simulink library "r2daq_blocks"  (R2012b)
settings: Solver=ode45  StartTime=0.0  StopTime=10.0  RelTol=1e-3
undefined symbols (not defined in the file or in its folder): biquad_iir, feedback_iir, filters, libddc, sfp, synth, xlfir_8x16
libraries: xbsIndex_r4 x4088, casper_library_misc x21, dspsigops x16, casper_library_delays x10, xps_library x1
(part 4 of 23)

== system r2daq_blocks/DigitalDownConverterExt/bus_mul_sine ==
  a : Inport
  b : Inport  Port=2
  a*b_bussify : Subsystem  AncestorBlock=casper_library_flow_control/bus_create  mask(bus_create){inputNum=16}
      mask prompts: inputNum "Number of inputs:"
      mask init:
      | bus_create_init(gcb,...
      |     'inputNum', inputNum);
  a_debus : Subsystem  AncestorBlock=casper_library_flow_control/bus_expand  mask(bus_expand){mode=divisions of arbitrary size, outputNum=1, outputWidth=[8 8 8 8 8 8 8 8 8 8 8 8 8 8 8 8], outputBinaryPt=[7 7 7 7 7 7 7 7 7 7 7 7 7 7 7 7], outputArithmeticType=[1 1 1 1 1 1 1 1 1 1 1 1 1 1 1 1], show_format=on, outputToWorkspace=off, variablePrefix=, outputToModelAsWell=on}
      mask prompts: outputNum "Number of outputs:"; outputWidth "Output width [msb ... lsb]:"; outputBinaryPt "Output binary point position [msb ... lsb]:"; outputArithmeticType "Output arithmetic type (ufix=0, fix=1, bool=2) [msb ... lsb]:"; show_format "Print format string?"; outputToWorkspace "Output to workspace?"; variablePrefix "Variable name prefix:"; outputToModelAsWell "Output to model as well?"
      mask help:
      | Expands a 'bus' made using a bus_create or Xilinx
      | concat block.
      | The input will be divided into the specified number
      | of outputs with the specified arithmetic types.
      | Divisions are made from most significant bit.
      mask init: same as r2daq_blocks/DigitalDownConverterExt/bus_mul_cosine/a_debus
      settings: AttributesFormatString=16 outputs: f8.7,f8.7,f8.7,f8.7,f8.7,f8.7,f8.7,f8.7,f8.7,f8.7,f8.7,f8.7,f8.7,f8.7,f8.7,f8.7,
      mask TypeOptions mode: divisions of equal size | divisions of arbitrary size
      mask Callback mode: bus_expand_callback();
      mask Callback outputWidth: bus_expand_callback();
      mask Callback outputToWorkspace: bus_expand_callback();
  b_debus : Subsystem  AncestorBlock=casper_library_flow_control/bus_expand  mask(bus_expand){mode=divisions of arbitrary size, outputNum=1, outputWidth=[11 11 11 11 11 11 11 11 11 11 11 11 11 11 11 11], outputBinaryPt=[9 9 9 9 9 9 9 9 9 9 9 9 9 9 9 9], outputArithmeticType=[1 1 1 1 1 1 1 1 1 1 1 1 1 1 1 1], show_format=on, outputToWorkspace=off, variablePrefix=, outputToModelAsWell=on}
      mask prompts: outputNum "Number of outputs:"; outputWidth "Output width [msb ... lsb]:"; outputBinaryPt "Output binary point position [msb ... lsb]:"; outputArithmeticType "Output arithmetic type (ufix=0, fix=1, bool=2) [msb ... lsb]:"; show_format "Print format string?"; outputToWorkspace "Output to workspace?"; variablePrefix "Variable name prefix:"; outputToModelAsWell "Output to model as well?"
      mask help:
      | Expands a 'bus' made using a bus_create or Xilinx
      | concat block.
      | The input will be divided into the specified number
      | of outputs with the specified arithmetic types.
      | Divisions are made from most significant bit.
      mask init: same as r2daq_blocks/DigitalDownConverterExt/bus_mul_cosine/a_debus
      settings: AttributesFormatString=16 outputs: f11.9,f11.9,f11.9,f11.9,f11.9,f11.9,f11.9,f11.9,f11.9,f11.9,f11.9,f11.9,f11.9,f11.9,f11.9,f11.9,
      mask TypeOptions mode: divisions of equal size | divisions of arbitrary size
      mask Callback mode: bus_expand_callback();
      mask Callback outputWidth: bus_expand_callback();
      mask Callback outputToWorkspace: bus_expand_callback();
  mult{1..16} (16 alike) : xbsIndex_r4/Mult  precision=User Defined  arith_type="Signed  (2's comp)"  n_bits=18  bin_pt=16  quantization=Truncate  overflow=Wrap  en=off  latency=mult_latency  dbl_ovrd=off  use_behavioral_HDL=on  opt=Speed  use_embedded=off  optimum_pipeline=off  pipeline=on  use_rpm=on  placement_style=Triangular  block_type=mult
  repa : Subsystem  AncestorBlock=casper_library_bus/bus_replicate  mask(bus_replicate){replication=1, latency=0, misc=off, implementation=core}
      mask prompts: replication "replication factor"; misc "misc support"; implementation "delay implementation"
      mask help: Output bus formed by replicating input bus a number of times
      mask init:
      | bus_replicate_init(gcb, ...
      |     'replication', replication, ...
      |     'latency', latency, ...
      |     'implementation', implementation, ...
      |     'misc', misc);
      mask TypeOptions implementation: core | behavioral
  repb : Subsystem  AncestorBlock=casper_library_bus/bus_replicate  mask(bus_replicate){replication=1, latency=0, misc=off, implementation=core}
      mask prompts: replication "replication factor"; misc "misc support"; implementation "delay implementation"
      mask help: Output bus formed by replicating input bus a number of times
      mask init:
      | bus_replicate_init(gcb, ...
      |     'replication', replication, ...
      |     'latency', latency, ...
      |     'implementation', implementation, ...
      |     'misc', misc);
      mask TypeOptions implementation: core | behavioral
  a*b : Outport
  wires:
  a/1 -> repa/1(in)
  b/1 -> repb/1(in)
  repa/1(out) -> a_debus/1(bus_in)
  repb/1(out) -> b_debus/1(bus_in)
  a_debus/1(msb_out16) -> mult1/1
  b_debus/1(msb_out16) -> mult1/2
  a_debus/2(out15) -> mult2/1
  b_debus/2(out15) -> mult2/2
  a_debus/3(out14) -> mult3/1
  b_debus/3(out14) -> mult3/2
  a_debus/4(out13) -> mult4/1
  b_debus/4(out13) -> mult4/2
  a_debus/5(out12) -> mult5/1
  b_debus/5(out12) -> mult5/2
  a_debus/6(out11) -> mult6/1
  b_debus/6(out11) -> mult6/2
  a_debus/7(out10) -> mult7/1
  b_debus/7(out10) -> mult7/2
  a_debus/8(out9) -> mult8/1
  b_debus/8(out9) -> mult8/2
  a_debus/9(out8) -> mult9/1
  b_debus/9(out8) -> mult9/2
  a_debus/10(out7) -> mult10/1
  b_debus/10(out7) -> mult10/2
  a_debus/11(out6) -> mult11/1
  b_debus/11(out6) -> mult11/2
  a_debus/12(out5) -> mult12/1
  b_debus/12(out5) -> mult12/2
  a_debus/13(out4) -> mult13/1
  b_debus/13(out4) -> mult13/2
  a_debus/14(out3) -> mult14/1
  b_debus/14(out3) -> mult14/2
  a_debus/15(out2) -> mult15/1
  b_debus/15(out2) -> mult15/2
  a_debus/16(lsb_out1) -> mult16/1
  b_debus/16(lsb_out1) -> mult16/2
  mult1/1 -> a*b_bussify/1(in1)
  mult2/1 -> a*b_bussify/2(in2)
  mult3/1 -> a*b_bussify/3(in3)
  mult4/1 -> a*b_bussify/4(in4)
  mult5/1 -> a*b_bussify/5(in5)
  mult6/1 -> a*b_bussify/6(in6)
  mult7/1 -> a*b_bussify/7(in7)
  mult8/1 -> a*b_bussify/8(in8)
  mult9/1 -> a*b_bussify/9(in9)
  mult10/1 -> a*b_bussify/10(in10)
  mult11/1 -> a*b_bussify/11(in11)
  mult12/1 -> a*b_bussify/12(in12)
  mult13/1 -> a*b_bussify/13(in13)
  mult14/1 -> a*b_bussify/14(in14)
  mult15/1 -> a*b_bussify/15(in15)
  mult16/1 -> a*b_bussify/16(in16)
  a*b_bussify/1(bus_out) -> a*b/1

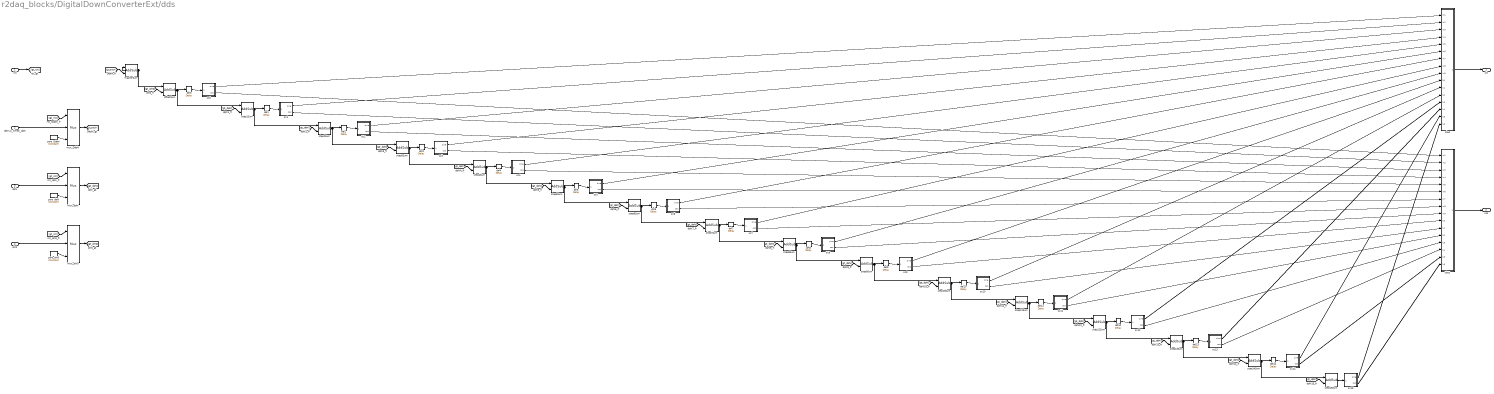
== system r2daq_blocks/DigitalDownConverterExt/dds ==
  rst : Inport
  demux_times_dphi : Inport  Port=2
  dphi : Inport  Port=3
  phi0 : Inport  Port=4
  cbus : Subsystem  AncestorBlock=casper_library_flow_control/bus_create  mask(bus_create){inputNum=16}
      mask prompts: inputNum "Number of inputs:"
      mask init:
      | bus_create_init(gcb,...
      |     'inputNum', inputNum);
  del0 : xbsIndex_r4/Delay  rst=off  infoeditControl=Selection of Reset will increase slice count due to use of real FFs and instead of SRLs  en=off  latency=15  dbl_ovrd=off  reg_retiming=off  block_type=delay
  del1 : xbsIndex_r4/Delay  rst=off  infoeditControl=Selection of Reset will increase slice count due to use of real FFs and instead of SRLs  en=off  latency=14  dbl_ovrd=off  reg_retiming=off  block_type=delay
  del10 : xbsIndex_r4/Delay  rst=off  infoeditControl=Selection of Reset will increase slice count due to use of real FFs and instead of SRLs  en=off  latency=5  dbl_ovrd=off  reg_retiming=off  block_type=delay
  del11 : xbsIndex_r4/Delay  rst=off  infoeditControl=Selection of Reset will increase slice count due to use of real FFs and instead of SRLs  en=off  latency=4  dbl_ovrd=off  reg_retiming=off  block_type=delay
  del12 : xbsIndex_r4/Delay  rst=off  infoeditControl=Selection of Reset will increase slice count due to use of real FFs and instead of SRLs  en=off  latency=3  dbl_ovrd=off  reg_retiming=off  block_type=delay
  del13 : xbsIndex_r4/Delay  rst=off  infoeditControl=Selection of Reset will increase slice count due to use of real FFs and instead of SRLs  en=off  latency=2  dbl_ovrd=off  reg_retiming=off  block_type=delay
  del14 : xbsIndex_r4/Delay  rst=off  infoeditControl=Selection of Reset will increase slice count due to use of real FFs and instead of SRLs  en=off  latency=1  dbl_ovrd=off  reg_retiming=off  block_type=delay
  del2 : xbsIndex_r4/Delay  rst=off  infoeditControl=Selection of Reset will increase slice count due to use of real FFs and instead of SRLs  en=off  latency=13  dbl_ovrd=off  reg_retiming=off  block_type=delay
  del3 : xbsIndex_r4/Delay  rst=off  infoeditControl=Selection of Reset will increase slice count due to use of real FFs and instead of SRLs  en=off  latency=12  dbl_ovrd=off  reg_retiming=off  block_type=delay
  del4 : xbsIndex_r4/Delay  rst=off  infoeditControl=Selection of Reset will increase slice count due to use of real FFs and instead of SRLs  en=off  latency=11  dbl_ovrd=off  reg_retiming=off  block_type=delay
  del5 : xbsIndex_r4/Delay  rst=off  infoeditControl=Selection of Reset will increase slice count due to use of real FFs and instead of SRLs  en=off  latency=10  dbl_ovrd=off  reg_retiming=off  block_type=delay
  del6 : xbsIndex_r4/Delay  rst=off  infoeditControl=Selection of Reset will increase slice count due to use of real FFs and instead of SRLs  en=off  latency=9  dbl_ovrd=off  reg_retiming=off  block_type=delay
  del7 : xbsIndex_r4/Delay  rst=off  infoeditControl=Selection of Reset will increase slice count due to use of real FFs and instead of SRLs  en=off  latency=8  dbl_ovrd=off  reg_retiming=off  block_type=delay
  del8 : xbsIndex_r4/Delay  rst=off  infoeditControl=Selection of Reset will increase slice count due to use of real FFs and instead of SRLs  en=off  latency=7  dbl_ovrd=off  reg_retiming=off  block_type=delay
  del9 : xbsIndex_r4/Delay  rst=off  infoeditControl=Selection of Reset will increase slice count due to use of real FFs and instead of SRLs  en=off  latency=6  dbl_ovrd=off  reg_retiming=off  block_type=delay
  masterSum : xbsIndex_r4/AddSub  mode=Addition  use_carryin=off  use_carryout=off  en=off  latency=1  precision=User Defined  arith_type=Unsigned  n_bits=10  bin_pt=0  quantization=Truncate  overflow=Wrap  dbl_ovrd=off  use_behavioral_HDL=off  hw_selection=Fabric  pipelined=off  block_type=addsub
  mux_Ddphi : xbsIndex_r4/Mux  inputs=2  en=off  latency=0  precision=Full  arith_type=Unsigned  n_bits=16  bin_pt=14  quantization=Truncate  overflow=Wrap  dbl_ovrd=off  block_type=mux
  mux_dphi : xbsIndex_r4/Mux  inputs=2  en=off  latency=0  precision=Full  arith_type=Unsigned  n_bits=16  bin_pt=14  quantization=Truncate  overflow=Wrap  dbl_ovrd=off  block_type=mux
  mux_phi0 : xbsIndex_r4/Mux  inputs=2  en=off  latency=0  precision=Full  arith_type=Unsigned  n_bits=16  bin_pt=14  quantization=Truncate  overflow=Wrap  dbl_ovrd=off  block_type=mux
  offsetSum : xbsIndex_r4/AddSub  mode=Addition  use_carryin=off  use_carryout=off  en=off  latency=1  precision=User Defined  arith_type=Unsigned  n_bits=10  bin_pt=0  quantization=Truncate  overflow=Wrap  dbl_ovrd=off  use_behavioral_HDL=off  hw_selection=Fabric  pipelined=off  block_type=addsub
  sbus : Subsystem  AncestorBlock=casper_library_flow_control/bus_create  mask(bus_create){inputNum=16}
      mask prompts: inputNum "Number of inputs:"
      mask init:
      | bus_create_init(gcb,...
      |     'inputNum', inputNum);
  sc0 : Subsystem  Tag=casper:sincos  AncestorBlock=casper_library_downconverter/sincos  mask(sincos){func=sine and cosine, neg_sin=off, neg_cos=off, symmetric=on, handle_sync=off, depth_bits=10, bit_width=11, bram_latency=2}
      mask prompts: func "Function"; neg_sin "Negative sine"; neg_cos "Negative cosine"; symmetric "Symmetric output"; handle_sync "Handle sync"; depth_bits "Lookup table depth (2^?)"; bit_width "Output bit width"; bram_latency "BRAM latency"
      mask init:
      | sincos_init(gcb, ...
      |     'func', func, ...
      |     'neg_sin', neg_sin, ...
      |     'neg_cos', neg_cos, ...
      |     'symmetric', symmetric, ...
      |     'handle_sync', handle_sync, ...
      |     'depth_bits', depth_bits, ...
      |     'bit_width', bit_width, ...
      |     'bram_latency', bram_latency);
      mask TypeOptions func: cosine | sine | sine and cosine
  sc1 : Subsystem  Tag=casper:sincos  AncestorBlock=casper_library_downconverter/sincos  mask(sincos){func=sine and cosine, neg_sin=off, neg_cos=off, symmetric=on, handle_sync=off, depth_bits=10, bit_width=11, bram_latency=2}
      mask prompts: func "Function"; neg_sin "Negative sine"; neg_cos "Negative cosine"; symmetric "Symmetric output"; handle_sync "Handle sync"; depth_bits "Lookup table depth (2^?)"; bit_width "Output bit width"; bram_latency "BRAM latency"
      mask init: same as r2daq_blocks/DigitalDownConverterExt/dds/sc0
      mask TypeOptions func: cosine | sine | sine and cosine
  sc10 : Subsystem  Tag=casper:sincos  AncestorBlock=casper_library_downconverter/sincos  mask(sincos){func=sine and cosine, neg_sin=off, neg_cos=off, symmetric=on, handle_sync=off, depth_bits=10, bit_width=11, bram_latency=2}
      mask prompts: func "Function"; neg_sin "Negative sine"; neg_cos "Negative cosine"; symmetric "Symmetric output"; handle_sync "Handle sync"; depth_bits "Lookup table depth (2^?)"; bit_width "Output bit width"; bram_latency "BRAM latency"
      mask init: same as r2daq_blocks/DigitalDownConverterExt/dds/sc0
      mask TypeOptions func: cosine | sine | sine and cosine
  sc11 : Subsystem  Tag=casper:sincos  AncestorBlock=casper_library_downconverter/sincos  mask(sincos){func=sine and cosine, neg_sin=off, neg_cos=off, symmetric=on, handle_sync=off, depth_bits=10, bit_width=11, bram_latency=2}
      mask prompts: func "Function"; neg_sin "Negative sine"; neg_cos "Negative cosine"; symmetric "Symmetric output"; handle_sync "Handle sync"; depth_bits "Lookup table depth (2^?)"; bit_width "Output bit width"; bram_latency "BRAM latency"
      mask init: same as r2daq_blocks/DigitalDownConverterExt/dds/sc0
      mask TypeOptions func: cosine | sine | sine and cosine
  sc12 : Subsystem  Tag=casper:sincos  AncestorBlock=casper_library_downconverter/sincos  mask(sincos){func=sine and cosine, neg_sin=off, neg_cos=off, symmetric=on, handle_sync=off, depth_bits=10, bit_width=11, bram_latency=2}
      mask prompts: func "Function"; neg_sin "Negative sine"; neg_cos "Negative cosine"; symmetric "Symmetric output"; handle_sync "Handle sync"; depth_bits "Lookup table depth (2^?)"; bit_width "Output bit width"; bram_latency "BRAM latency"
      mask init: same as r2daq_blocks/DigitalDownConverterExt/dds/sc0
      mask TypeOptions func: cosine | sine | sine and cosine
  sc13 : Subsystem  Tag=casper:sincos  AncestorBlock=casper_library_downconverter/sincos  mask(sincos){func=sine and cosine, neg_sin=off, neg_cos=off, symmetric=on, handle_sync=off, depth_bits=10, bit_width=11, bram_latency=2}
      mask prompts: func "Function"; neg_sin "Negative sine"; neg_cos "Negative cosine"; symmetric "Symmetric output"; handle_sync "Handle sync"; depth_bits "Lookup table depth (2^?)"; bit_width "Output bit width"; bram_latency "BRAM latency"
      mask init: same as r2daq_blocks/DigitalDownConverterExt/dds/sc0
      mask TypeOptions func: cosine | sine | sine and cosine
  sc14 : Subsystem  Tag=casper:sincos  AncestorBlock=casper_library_downconverter/sincos  mask(sincos){func=sine and cosine, neg_sin=off, neg_cos=off, symmetric=on, handle_sync=off, depth_bits=10, bit_width=11, bram_latency=2}
      mask prompts: func "Function"; neg_sin "Negative sine"; neg_cos "Negative cosine"; symmetric "Symmetric output"; handle_sync "Handle sync"; depth_bits "Lookup table depth (2^?)"; bit_width "Output bit width"; bram_latency "BRAM latency"
      mask init: same as r2daq_blocks/DigitalDownConverterExt/dds/sc0
      mask TypeOptions func: cosine | sine | sine and cosine
  sc15 : Subsystem  Tag=casper:sincos  AncestorBlock=casper_library_downconverter/sincos  mask(sincos){func=sine and cosine, neg_sin=off, neg_cos=off, symmetric=on, handle_sync=off, depth_bits=10, bit_width=11, bram_latency=2}
      mask prompts: func "Function"; neg_sin "Negative sine"; neg_cos "Negative cosine"; symmetric "Symmetric output"; handle_sync "Handle sync"; depth_bits "Lookup table depth (2^?)"; bit_width "Output bit width"; bram_latency "BRAM latency"
      mask init: same as r2daq_blocks/DigitalDownConverterExt/dds/sc0
      mask TypeOptions func: cosine | sine | sine and cosine
  sc2 : Subsystem  Tag=casper:sincos  AncestorBlock=casper_library_downconverter/sincos  mask(sincos){func=sine and cosine, neg_sin=off, neg_cos=off, symmetric=on, handle_sync=off, depth_bits=10, bit_width=11, bram_latency=2}
      mask prompts: func "Function"; neg_sin "Negative sine"; neg_cos "Negative cosine"; symmetric "Symmetric output"; handle_sync "Handle sync"; depth_bits "Lookup table depth (2^?)"; bit_width "Output bit width"; bram_latency "BRAM latency"
      mask init: same as r2daq_blocks/DigitalDownConverterExt/dds/sc0
      mask TypeOptions func: cosine | sine | sine and cosine
  sc3 : Subsystem  Tag=casper:sincos  AncestorBlock=casper_library_downconverter/sincos  mask(sincos){func=sine and cosine, neg_sin=off, neg_cos=off, symmetric=on, handle_sync=off, depth_bits=10, bit_width=11, bram_latency=2}
      mask prompts: func "Function"; neg_sin "Negative sine"; neg_cos "Negative cosine"; symmetric "Symmetric output"; handle_sync "Handle sync"; depth_bits "Lookup table depth (2^?)"; bit_width "Output bit width"; bram_latency "BRAM latency"
      mask init: same as r2daq_blocks/DigitalDownConverterExt/dds/sc0
      mask TypeOptions func: cosine | sine | sine and cosine
  sc4 : Subsystem  Tag=casper:sincos  AncestorBlock=casper_library_downconverter/sincos  mask(sincos){func=sine and cosine, neg_sin=off, neg_cos=off, symmetric=on, handle_sync=off, depth_bits=10, bit_width=11, bram_latency=2}
      mask prompts: func "Function"; neg_sin "Negative sine"; neg_cos "Negative cosine"; symmetric "Symmetric output"; handle_sync "Handle sync"; depth_bits "Lookup table depth (2^?)"; bit_width "Output bit width"; bram_latency "BRAM latency"
      mask init: same as r2daq_blocks/DigitalDownConverterExt/dds/sc0
      mask TypeOptions func: cosine | sine | sine and cosine
  sc5 : Subsystem  Tag=casper:sincos  AncestorBlock=casper_library_downconverter/sincos  mask(sincos){func=sine and cosine, neg_sin=off, neg_cos=off, symmetric=on, handle_sync=off, depth_bits=10, bit_width=11, bram_latency=2}
      mask prompts: func "Function"; neg_sin "Negative sine"; neg_cos "Negative cosine"; symmetric "Symmetric output"; handle_sync "Handle sync"; depth_bits "Lookup table depth (2^?)"; bit_width "Output bit width"; bram_latency "BRAM latency"
      mask init: same as r2daq_blocks/DigitalDownConverterExt/dds/sc0
      mask TypeOptions func: cosine | sine | sine and cosine
  sc6 : Subsystem  Tag=casper:sincos  AncestorBlock=casper_library_downconverter/sincos  mask(sincos){func=sine and cosine, neg_sin=off, neg_cos=off, symmetric=on, handle_sync=off, depth_bits=10, bit_width=11, bram_latency=2}
      mask prompts: func "Function"; neg_sin "Negative sine"; neg_cos "Negative cosine"; symmetric "Symmetric output"; handle_sync "Handle sync"; depth_bits "Lookup table depth (2^?)"; bit_width "Output bit width"; bram_latency "BRAM latency"
      mask init: same as r2daq_blocks/DigitalDownConverterExt/dds/sc0
      mask TypeOptions func: cosine | sine | sine and cosine
  sc7 : Subsystem  Tag=casper:sincos  AncestorBlock=casper_library_downconverter/sincos  mask(sincos){func=sine and cosine, neg_sin=off, neg_cos=off, symmetric=on, handle_sync=off, depth_bits=10, bit_width=11, bram_latency=2}
      mask prompts: func "Function"; neg_sin "Negative sine"; neg_cos "Negative cosine"; symmetric "Symmetric output"; handle_sync "Handle sync"; depth_bits "Lookup table depth (2^?)"; bit_width "Output bit width"; bram_latency "BRAM latency"
      mask init: same as r2daq_blocks/DigitalDownConverterExt/dds/sc0
      mask TypeOptions func: cosine | sine | sine and cosine
  sc8 : Subsystem  Tag=casper:sincos  AncestorBlock=casper_library_downconverter/sincos  mask(sincos){func=sine and cosine, neg_sin=off, neg_cos=off, symmetric=on, handle_sync=off, depth_bits=10, bit_width=11, bram_latency=2}
      mask prompts: func "Function"; neg_sin "Negative sine"; neg_cos "Negative cosine"; symmetric "Symmetric output"; handle_sync "Handle sync"; depth_bits "Lookup table depth (2^?)"; bit_width "Output bit width"; bram_latency "BRAM latency"
      mask init: same as r2daq_blocks/DigitalDownConverterExt/dds/sc0
      mask TypeOptions func: cosine | sine | sine and cosine
  sc9 : Subsystem  Tag=casper:sincos  AncestorBlock=casper_library_downconverter/sincos  mask(sincos){func=sine and cosine, neg_sin=off, neg_cos=off, symmetric=on, handle_sync=off, depth_bits=10, bit_width=11, bram_latency=2}
      mask prompts: func "Function"; neg_sin "Negative sine"; neg_cos "Negative cosine"; symmetric "Symmetric output"; handle_sync "Handle sync"; depth_bits "Lookup table depth (2^?)"; bit_width "Output bit width"; bram_latency "BRAM latency"
      mask init: same as r2daq_blocks/DigitalDownConverterExt/dds/sc0
      mask TypeOptions func: cosine | sine | sine and cosine
  step10Sum : xbsIndex_r4/AddSub  mode=Addition  use_carryin=off  use_carryout=off  en=off  latency=1  precision=User Defined  arith_type=Unsigned  n_bits=10  bin_pt=0  quantization=Truncate  overflow=Wrap  dbl_ovrd=off  use_behavioral_HDL=off  hw_selection=Fabric  pipelined=off  block_type=addsub
  step11Sum : xbsIndex_r4/AddSub  mode=Addition  use_carryin=off  use_carryout=off  en=off  latency=1  precision=User Defined  arith_type=Unsigned  n_bits=10  bin_pt=0  quantization=Truncate  overflow=Wrap  dbl_ovrd=off  use_behavioral_HDL=off  hw_selection=Fabric  pipelined=off  block_type=addsub
  step12Sum : xbsIndex_r4/AddSub  mode=Addition  use_carryin=off  use_carryout=off  en=off  latency=1  precision=User Defined  arith_type=Unsigned  n_bits=10  bin_pt=0  quantization=Truncate  overflow=Wrap  dbl_ovrd=off  use_behavioral_HDL=off  hw_selection=Fabric  pipelined=off  block_type=addsub
  step13Sum : xbsIndex_r4/AddSub  mode=Addition  use_carryin=off  use_carryout=off  en=off  latency=1  precision=User Defined  arith_type=Unsigned  n_bits=10  bin_pt=0  quantization=Truncate  overflow=Wrap  dbl_ovrd=off  use_behavioral_HDL=off  hw_selection=Fabric  pipelined=off  block_type=addsub
  step14Sum : xbsIndex_r4/AddSub  mode=Addition  use_carryin=off  use_carryout=off  en=off  latency=1  precision=User Defined  arith_type=Unsigned  n_bits=10  bin_pt=0  quantization=Truncate  overflow=Wrap  dbl_ovrd=off  use_behavioral_HDL=off  hw_selection=Fabric  pipelined=off  block_type=addsub
  step15Sum : xbsIndex_r4/AddSub  mode=Addition  use_carryin=off  use_carryout=off  en=off  latency=1  precision=User Defined  arith_type=Unsigned  n_bits=10  bin_pt=0  quantization=Truncate  overflow=Wrap  dbl_ovrd=off  use_behavioral_HDL=off  hw_selection=Fabric  pipelined=off  block_type=addsub
  step1Sum : xbsIndex_r4/AddSub  mode=Addition  use_carryin=off  use_carryout=off  en=off  latency=1  precision=User Defined  arith_type=Unsigned  n_bits=10  bin_pt=0  quantization=Truncate  overflow=Wrap  dbl_ovrd=off  use_behavioral_HDL=off  hw_selection=Fabric  pipelined=off  block_type=addsub
  step2Sum : xbsIndex_r4/AddSub  mode=Addition  use_carryin=off  use_carryout=off  en=off  latency=1  precision=User Defined  arith_type=Unsigned  n_bits=10  bin_pt=0  quantization=Truncate  overflow=Wrap  dbl_ovrd=off  use_behavioral_HDL=off  hw_selection=Fabric  pipelined=off  block_type=addsub
  step3Sum : xbsIndex_r4/AddSub  mode=Addition  use_carryin=off  use_carryout=off  en=off  latency=1  precision=User Defined  arith_type=Unsigned  n_bits=10  bin_pt=0  quantization=Truncate  overflow=Wrap  dbl_ovrd=off  use_behavioral_HDL=off  hw_selection=Fabric  pipelined=off  block_type=addsub
  step4Sum : xbsIndex_r4/AddSub  mode=Addition  use_carryin=off  use_carryout=off  en=off  latency=1  precision=User Defined  arith_type=Unsigned  n_bits=10  bin_pt=0  quantization=Truncate  overflow=Wrap  dbl_ovrd=off  use_behavioral_HDL=off  hw_selection=Fabric  pipelined=off  block_type=addsub
  step5Sum : xbsIndex_r4/AddSub  mode=Addition  use_carryin=off  use_carryout=off  en=off  latency=1  precision=User Defined  arith_type=Unsigned  n_bits=10  bin_pt=0  quantization=Truncate  overflow=Wrap  dbl_ovrd=off  use_behavioral_HDL=off  hw_selection=Fabric  pipelined=off  block_type=addsub
  step6Sum : xbsIndex_r4/AddSub  mode=Addition  use_carryin=off  use_carryout=off  en=off  latency=1  precision=User Defined  arith_type=Unsigned  n_bits=10  bin_pt=0  quantization=Truncate  overflow=Wrap  dbl_ovrd=off  use_behavioral_HDL=off  hw_selection=Fabric  pipelined=off  block_type=addsub
  step7Sum : xbsIndex_r4/AddSub  mode=Addition  use_carryin=off  use_carryout=off  en=off  latency=1  precision=User Defined  arith_type=Unsigned  n_bits=10  bin_pt=0  quantization=Truncate  overflow=Wrap  dbl_ovrd=off  use_behavioral_HDL=off  hw_selection=Fabric  pipelined=off  block_type=addsub
  step8Sum : xbsIndex_r4/AddSub  mode=Addition  use_carryin=off  use_carryout=off  en=off  latency=1  precision=User Defined  arith_type=Unsigned  n_bits=10  bin_pt=0  quantization=Truncate  overflow=Wrap  dbl_ovrd=off  use_behavioral_HDL=off  hw_selection=Fabric  pipelined=off  block_type=addsub
  step9Sum : xbsIndex_r4/AddSub  mode=Addition  use_carryin=off  use_carryout=off  en=off  latency=1  precision=User Defined  arith_type=Unsigned  n_bits=10  bin_pt=0  quantization=Truncate  overflow=Wrap  dbl_ovrd=off  use_behavioral_HDL=off  hw_selection=Fabric  pipelined=off  block_type=addsub
  zero_Ddphi : xbsIndex_r4/Constant  const=0  gui_display_data_type=Fixed-point  arith_type=Unsigned  n_bits=10  bin_pt=0  preci_type=Single  exp_width=8  frac_width=24  explicit_period=on  period=1  equ=P=C  opselect=C  inp2=PCIN>>17  opr=+  inp1=P  carry=CIN  dbl_ovrd=off  block_type=constant
  zero_dphi : xbsIndex_r4/Constant  const=0  gui_display_data_type=Fixed-point  arith_type=Unsigned  n_bits=10  bin_pt=0  preci_type=Single  exp_width=8  frac_width=24  explicit_period=on  period=1  equ=P=C  opselect=C  inp2=PCIN>>17  opr=+  inp1=P  carry=CIN  dbl_ovrd=off  block_type=constant
  zero_phi0 : xbsIndex_r4/Constant  const=0  gui_display_data_type=Fixed-point  arith_type=Unsigned  n_bits=10  bin_pt=0  preci_type=Single  exp_width=8  frac_width=24  explicit_period=on  period=1  equ=P=C  opselect=C  inp2=PCIN>>17  opr=+  inp1=P  carry=CIN  dbl_ovrd=off  block_type=constant
  sin : Outport
  cos : Outport  Port=2
  wires:
  rst/1 -> [gt_rst]
  [gt_rst] -> mux_Ddphi/1
  zero_Ddphi/1 -> mux_Ddphi/3
  demux_times_dphi/1 -> mux_Ddphi/2
  [gt_rst] -> mux_dphi/1
  zero_dphi/1 -> mux_dphi/3
  dphi/1 -> mux_dphi/2
  [gt_rst] -> mux_phi0/1
  zero_phi0/1 -> mux_phi0/3
  phi0/1 -> mux_phi0/2
  mux_Ddphi/1 -> [gt_Ddphi]
  mux_dphi/1 -> [gt_dphi]
  mux_phi0/1 -> [gt_phi0]
  [gt_Ddphi] -> masterSum/2
  masterSum/1 -> masterSum/1, offsetSum/1
  [gt_phi0] -> offsetSum/2
  offsetSum/1 -> del0/1, step1Sum/1
  del0/1 -> sc0/1(theta)
  [gt_dphi] -> step1Sum/2
  step1Sum/1 -> del1/1, step2Sum/1
  del1/1 -> sc1/1(theta)
  [gt_dphi] -> step2Sum/2
  step2Sum/1 -> del2/1, step3Sum/1
  del2/1 -> sc2/1(theta)
  [gt_dphi] -> step3Sum/2
  step3Sum/1 -> del3/1, step4Sum/1
  del3/1 -> sc3/1(theta)
  [gt_dphi] -> step4Sum/2
  step4Sum/1 -> del4/1, step5Sum/1
  del4/1 -> sc4/1(theta)
  [gt_dphi] -> step5Sum/2
  step5Sum/1 -> del5/1, step6Sum/1
  del5/1 -> sc5/1(theta)
  [gt_dphi] -> step6Sum/2
  step6Sum/1 -> del6/1, step7Sum/1
  del6/1 -> sc6/1(theta)
  [gt_dphi] -> step7Sum/2
  step7Sum/1 -> del7/1, step8Sum/1
  del7/1 -> sc7/1(theta)
  [gt_dphi] -> step8Sum/2
  step8Sum/1 -> del8/1, step9Sum/1
  del8/1 -> sc8/1(theta)
  [gt_dphi] -> step9Sum/2
  step9Sum/1 -> del9/1, step10Sum/1
  del9/1 -> sc9/1(theta)
  [gt_dphi] -> step10Sum/2
  step10Sum/1 -> del10/1, step11Sum/1
  del10/1 -> sc10/1(theta)
  [gt_dphi] -> step11Sum/2
  step11Sum/1 -> del11/1, step12Sum/1
  del11/1 -> sc11/1(theta)
  [gt_dphi] -> step12Sum/2
  step12Sum/1 -> del12/1, step13Sum/1
  del12/1 -> sc12/1(theta)
  [gt_dphi] -> step13Sum/2
  step13Sum/1 -> del13/1, step14Sum/1
  del13/1 -> sc13/1(theta)
  [gt_dphi] -> step14Sum/2
  step14Sum/1 -> del14/1, step15Sum/1
  del14/1 -> sc14/1(theta)
  [gt_dphi] -> step15Sum/2
  step15Sum/1 -> sc15/1(theta)
  sc0/1(sine) -> sbus/1(in1)
  sc1/1(sine) -> sbus/2(in2)
  sc2/1(sine) -> sbus/3(in3)
  sc3/1(sine) -> sbus/4(in4)
  sc4/1(sine) -> sbus/5(in5)
  sc5/1(sine) -> sbus/6(in6)
  sc6/1(sine) -> sbus/7(in7)
  sc7/1(sine) -> sbus/8(in8)
  sc8/1(sine) -> sbus/9(in9)
  sc9/1(sine) -> sbus/10(in10)
  sc10/1(sine) -> sbus/11(in11)
  sc11/1(sine) -> sbus/12(in12)
  sc12/1(sine) -> sbus/13(in13)
  sc13/1(sine) -> sbus/14(in14)
  sc14/1(sine) -> sbus/15(in15)
  sc15/1(sine) -> sbus/16(in16)
  sbus/1(bus_out) -> sin/1
  sc0/2(cos) -> cbus/1(in1)
  sc1/2(cos) -> cbus/2(in2)
  sc2/2(cos) -> cbus/3(in3)
  sc3/2(cos) -> cbus/4(in4)
  sc4/2(cos) -> cbus/5(in5)
  sc5/2(cos) -> cbus/6(in6)
  sc6/2(cos) -> cbus/7(in7)
  sc7/2(cos) -> cbus/8(in8)
  sc8/2(cos) -> cbus/9(in9)
  sc9/2(cos) -> cbus/10(in10)
  sc10/2(cos) -> cbus/11(in11)
  sc11/2(cos) -> cbus/12(in12)
  sc12/2(cos) -> cbus/13(in13)
  sc13/2(cos) -> cbus/14(in14)
  sc14/2(cos) -> cbus/15(in15)
  sc15/2(cos) -> cbus/16(in16)
  cbus/1(bus_out) -> cos/1
